simulink model "model"  (R2023a)
settings: Solver=VariableStepAuto  StartTime=0.0  StopTime=10.0  RelTol=1e-3
values from neighbouring files (symbols this model uses):
  K = real(K)    [solveKMatrix.m]
settings Model: Creator=Carson  LastModifiedBy=Carson

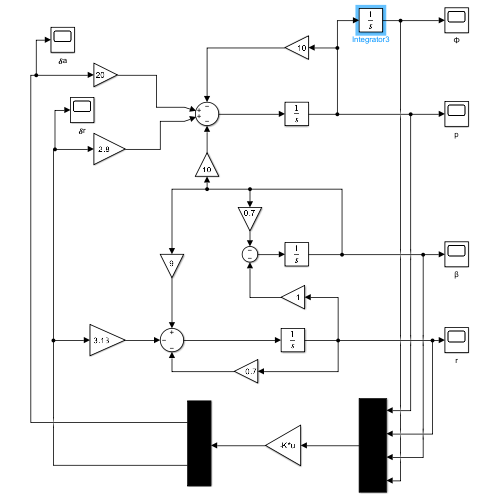
[thumbnail: Simulink's stored preview of the top-level diagram]
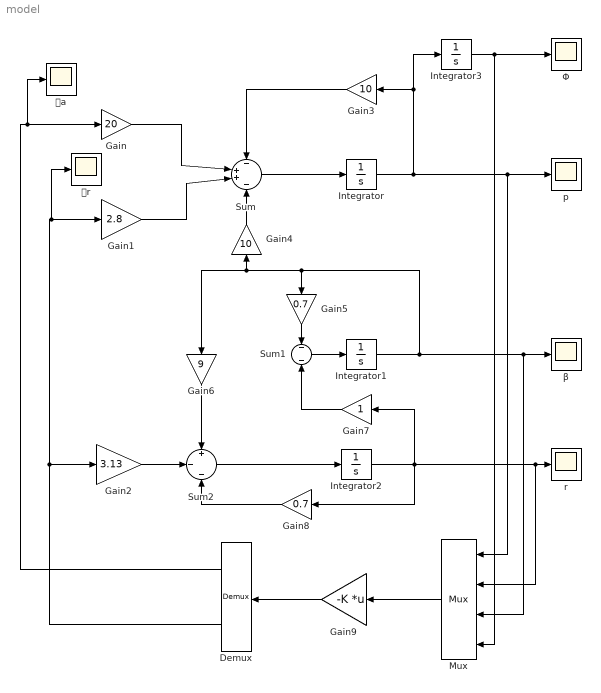
== system model ==
  Demux : Demux  Outputs=2
  Gain : Gain  Gain=20
  Gain1 : Gain  Gain=2.8
  Gain2 : Gain  Gain=3.13
  Gain3 : Gain  Gain=10
  Gain4 : Gain  Gain=10
  Gain5 : Gain  Gain=0.7
  Gain6 : Gain  Gain=9
  Gain7 : Gain
  Gain8 : Gain  Gain=0.7
  Gain9 : Gain  Gain=-K  Multiplication=Matrix(K*u)
  Integrator : Integrator
  Integrator1 : Integrator
  Integrator2 : Integrator
  Integrator3 : Integrator  InitialCondition=0.5236
  Mux : Mux
  Sum : Sum  Inputs=-|++|-
  Sum1 : Sum  Inputs=-||-
  Sum2 : Sum  Inputs=+|-|-
  p : Scope
  r : Scope
  Φ : Scope
  β : Scope
  𝜹a : Scope
  𝜹r : Scope
  wires:
  Integrator/1 -> Integrator3/1, Gain3/1, Mux/1, p/1
  Integrator1/1 -> Mux/3, β/1, Gain6/1, Gain4/1, Gain5/1
  Integrator2/1 -> Gain8/1, Gain7/1, Mux/2, r/1
  Gain/1 -> Sum/2
  Gain3/1 -> Sum/1
  Sum/1 -> Integrator/1
  Gain1/1 -> Sum/3
  Gain4/1 -> Sum/4
  Sum2/1 -> Integrator2/1
  Sum1/1 -> Integrator1/1
  Gain5/1 -> Sum1/1
  Gain2/1 -> Sum2/2
  Gain6/1 -> Sum2/1
  Gain7/1 -> Sum1/2
  Gain8/1 -> Sum2/3
  Integrator3/1 -> Mux/4, Φ/1
  Mux/1 -> Gain9/1
  Gain9/1 -> Demux/1
  Demux/1 -> 𝜹a/1, Gain/1
  Demux/2 -> Gain2/1, 𝜹r/1, Gain1/1
